simulink model "Aufgabe2d_sim"  (R2023b)
settings: Solver=VariableStepAuto  StartTime=0.0  StopTime=10.0  RelTol=1e-3
values from neighbouring files (symbols this model uses):
  gewicht = 0    [Aufgabe2d_param.m]
  K1 = 1    [Aufgabe2d_param.m]
  K2 = 1    [Aufgabe2d_param.m]
  K3 = 1    [Aufgabe2d_param.m]
  Kr = Kr_array(count)    [Aufgabe2d_param.m]
  T1 = 1e-3    (= 0.001)    [Aufgabe2d_param.m]
  T2 = 0.75e-3    (= 0.00075)    [Aufgabe2d_param.m]
  T3 = 0.5e-3    (= 0.0005)    [Aufgabe2d_param.m]
settings Model: Creator=Rouven Harmgarth  LastModifiedBy=Rouven Harmgarth

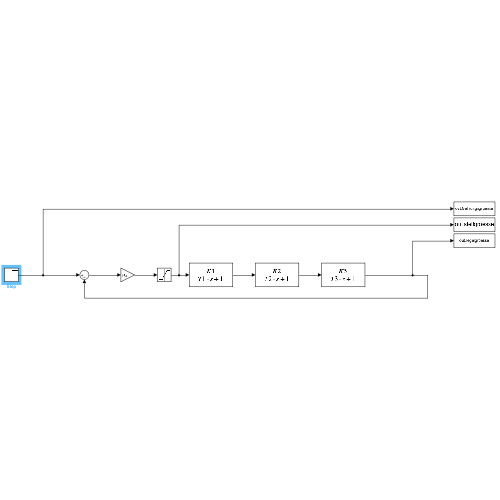
[thumbnail: Simulink's stored preview of the top-level diagram]
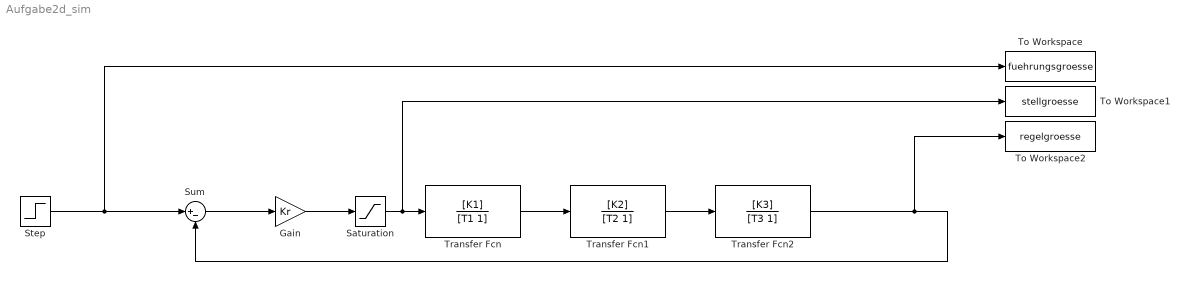
== system Aufgabe2d_sim ==
  Gain : Gain  Gain=Kr
  Saturation : Saturate  UpperLimit=12  LowerLimit=-12
  Step : Step  Time=0  After=gewicht  SampleTime=0
  Sum : Sum  Inputs=|+-
  To Workspace : ToWorkspace  VariableName=fuehrungsgroesse  SaveFormat=Structure With Time  SampleTime=-1
  To Workspace1 : ToWorkspace  VariableName=stellgroesse  SaveFormat=Structure With Time  SampleTime=-1
  To Workspace2 : ToWorkspace  VariableName=regelgroesse  SaveFormat=Structure With Time  SampleTime=-1
  Transfer Fcn : TransferFcn  Numerator=[K1]  Denominator=[T1 1]
  Transfer Fcn1 : TransferFcn  Numerator=[K2]  Denominator=[T2 1]
  Transfer Fcn2 : TransferFcn  Numerator=[K3]  Denominator=[T3 1]
  wires:
  Transfer Fcn/1 -> Transfer Fcn1/1
  Transfer Fcn1/1 -> Transfer Fcn2/1
  Saturation/1 -> To Workspace1/1, Transfer Fcn/1
  Gain/1 -> Saturation/1
  Sum/1 -> Gain/1
  Step/1 -> To Workspace/1, Sum/1
  Transfer Fcn2/1 -> To Workspace2/1, Sum/2
